simulink model "Copy_2_of_quad_drone"  (R2026a)
settings: Solver=ode4  StopTime=110
values from neighbouring files (symbols this model uses):
  accel_bias_init = [0.05; -0.03; 0.04]    [drone_params.m]    (also in new_drone_params.m)
  accel_drift_std = 0.0001    [drone_params.m]    (also in new_drone_params.m)
  accel_noise_std = 0.007    [drone_params.m]    (also in new_drone_params.m)
  circle_alt = -10    [drone_params.m]    (also in new_drone_params.m)
  circle_center_x = 0    [drone_params.m]    (also in new_drone_params.m)
  circle_center_y = 0    [drone_params.m]    (also in new_drone_params.m)
  circle_radius = 15    [drone_params.m]    (also in new_drone_params.m)
  circle_speed = 1.0    (= 1)    [drone_params.m]    (also in new_drone_params.m)
  g = 9.81    [drone_params.m]    (also in new_drone_params.m)
  gyro_bias_init = [0.002; -0.001; 0.003]    [drone_params.m]    (also in new_drone_params.m)
  gyro_drift_std = 0.0001    [drone_params.m]    (also in new_drone_params.m)
  gyro_noise_std = 0.005    [drone_params.m]    (also in new_drone_params.m)
  kD = 1.5e-7    (= 1.5e-07)    [drone_params.m]    (also in new_drone_params.m)
  Kd_att = [3.5; 3.5; 2]    [drone_params.m]    (also in new_drone_params.m)
  Kd_pos = [0.8; 1.2; 1.8]    [drone_params.m]    (also in new_drone_params.m)
  Kp_att = [6; 6; 4]    [drone_params.m]    (also in new_drone_params.m)
  Kp_pos = [0.5; 0.5; 1.0]    [drone_params.m]    (also in new_drone_params.m)
  kT = 1.2e-5    (= 1.2e-05)    [drone_params.m]    (also in new_drone_params.m)
  L = 0.25    [drone_params.m]    (also in new_drone_params.m; pnp_solver.m = pts_3d(i,:)')
  landmarks_3D = [city_landmarks; road_pts; light_pts; tree_pts; ground_pts]    [drone_params.m]    (also in initialize_map.m = zeros(500, 3); new_drone_params.m)
  m = 1.5    [drone_params.m]    (also in new_drone_params.m)
  num_landmarks = size(landmarks_3D, 1)    [drone_params.m]    (also in new_drone_params.m)
  P0 = K * [eye(3), zeros(3,1)]    [demo_vo_real_world.m]    (also in drone_params.m = diag([0.1, 0.1, 0.1,             0.1, 0.1, 0.1,             ; initialize_map.m; new_drone_params.m = diag([0.1, 0.1, 0.1,             0.1, 0.1, 0.1,             )
  Q_ekf = diag([1e-4, 1e-4, 1e-4,                1e-3, 1e-3, 1e-3,                1e-4, 1e-4, 1e-4,                1e-9, 1e-9, 1e-9,                1e-9, 1e-9, 1e-9])    [drone_params.m]    (also in new_drone_params.m)
  R_cam_body = [0 1 0; 0 0 1; 1 0 0]    [drone_params.m]    (also in generate_camera_frame.m; new_drone_params.m)
  R_ekf = diag([0.08^2, 0.08^2, 0.08^2,      0.05^2, 0.05^2, 0.05^2])    [drone_params.m]    (also in new_drone_params.m)
  takeoff_time = 12    [drone_params.m]    (also in new_drone_params.m)
  Ts = 0.001    [drone_params.m]    (also in new_drone_params.m)
  x0_ekf = Simulink.Parameter    [drone_params.m]
libraries: simulink x1, matrix_library x1
settings Model: Creator=Intern2  LastModifiedBy=Intern2
settings RTWCC: Toolchain=Microsoft Visual C++ 2022 v17.0 | nmake (64-bit Windows)

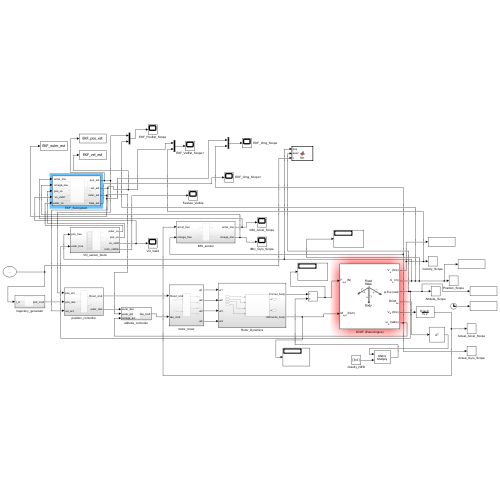
[thumbnail: Simulink's stored preview of the top-level diagram]
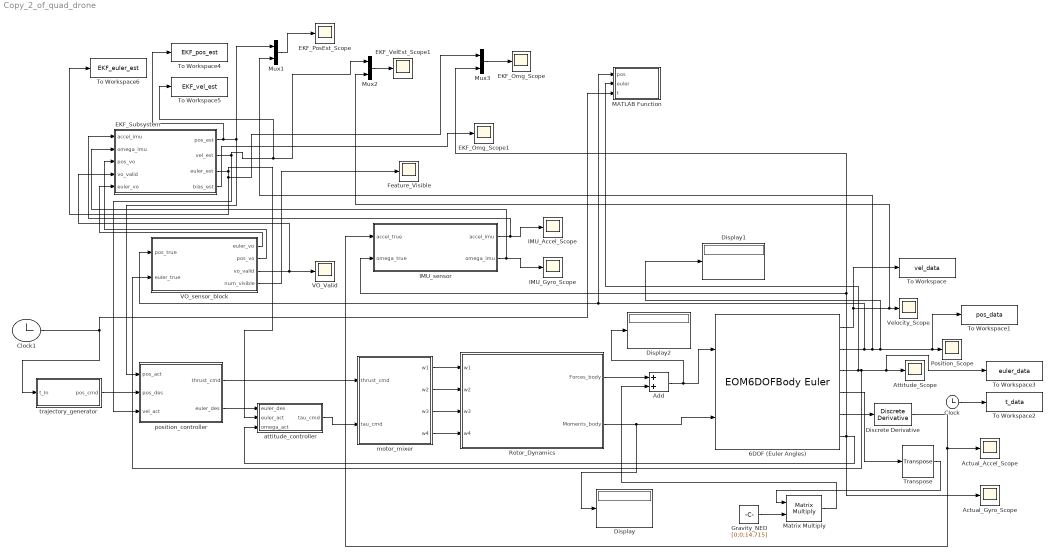
== system Copy_2_of_quad_drone ==
  6DOF (Euler Angles) : EOM6DOFBodyEuler  xme_0=pos_0  Vm_0=vel_0  eul_0=euler_0  pm_0=omega_0  mass_0=m  inertia=I_body
  Actual_Accel_Scope : Scope
      settings: ActiveDisplayYMinimum=-0.50165246590945589  ActiveDisplayYMaximum=0.65110460381560342  DataLoggingVariableName=ScopeData5
  Actual_Gyro_Scope : Scope
      settings: ActiveDisplayYMinimum=-0.42328851957372776  ActiveDisplayYMaximum=0.43797939700166927  DataLoggingVariableName=ScopeData6
  Add : Sum
  Attitude_Scope : Scope
      settings: ActiveDisplayYMinimum=-4.9243572148197217  ActiveDisplayYMaximum=6.6592750571240353  DataLoggingVariableName=ScopeData2
  Clock : Clock
  Clock1 : Clock
  Discrete Derivative : simulink/Discrete/Discrete Derivative  gainval=1.0  ICPrevScaledInput=0.0  OutMin=[]  OutMax=[]  OutDataType=fixdt(1, 16)  OutScaling=2^-10  DoSatur=off
  Display : Display
  Display1 : Display
  Display2 : Display
  EKF_Omg_Scope : Scope
      settings: ActiveDisplayYMinimum=-2.2293879743404958  ActiveDisplayYMaximum=4.7882717816873033  DataLoggingVariableName=ScopeData7
  EKF_Omg_Scope1 : Scope
      settings: ActiveDisplayYMinimum=-1.3068915384977462  ActiveDisplayYMaximum=2.7961887787070889  DataLoggingVariableName=ScopeData12
  EKF_PosEst_Scope : Scope
      settings: ActiveDisplayYMinimum=-40.340225147438069  ActiveDisplayYMaximum=49.360325650117439  DataLoggingVariableName=ScopeData10
  EKF_Subsystem : Subsystem
  EKF_VelEst_Scope1 : Scope
      settings: ActiveDisplayYMinimum=-3.7944004770804414  ActiveDisplayYMaximum=3.6966528557513043  DataLoggingVariableName=ScopeData11
  Feature_Visible : Scope
      settings: ActiveDisplayYMinimum=-641.958251221389  ActiveDisplayYMaximum=573.11142304309487  DataLoggingVariableName=ScopeData8
  Gravity_NED : Constant  Value=[0;0;14.715]
  IMU_Accel_Scope : Scope
      settings: ActiveDisplayYMinimum=-1.9727778311938033  ActiveDisplayYMaximum=2.0010412781388083  DataLoggingVariableName=ScopeData3
  IMU_Gyro_Scope : Scope
      settings: ActiveDisplayYMinimum=-0.092596809772179461  ActiveDisplayYMaximum=0.10856975643800111  DataLoggingVariableName=ScopeData4
  IMU_sensor : Subsystem
  MATLAB Function : MATLAB Function  TreatAsAtomicUnit=on
  Matrix Multiply : Product  Multiplication=Matrix(*)
  Mux1 : Mux  Inputs=2
  Mux2 : Mux  Inputs=2
  Mux3 : Mux  Inputs=2
  Position_Scope : Scope
      settings: ActiveDisplayYMinimum=-93.002014723178334  ActiveDisplayYMaximum=157.03895632222842
  Rotor_Dynamics : Subsystem
  To Workspace : ToWorkspace  VariableName=vel_data  SampleTime=-1
  To Workspace1 : ToWorkspace  VariableName=pos_data  SampleTime=-1
  To Workspace2 : ToWorkspace  VariableName=t_data  SampleTime=-1
  To Workspace3 : ToWorkspace  VariableName=euler_data  SampleTime=-1
  To Workspace4 : ToWorkspace  VariableName=EKF_pos_est  SampleTime=-1
  To Workspace5 : ToWorkspace  VariableName=EKF_vel_est  SampleTime=-1
  To Workspace6 : ToWorkspace  VariableName=EKF_euler_est  SampleTime=-1
  Transpose : matrix_library/Transpose
  VO_Valid : Scope
      settings: ActiveDisplayYMinimum=-4.4680085557439737  ActiveDisplayYMaximum=3.9129303872615759  DataLoggingVariableName=ScopeData9
  VO_sensor_block : Subsystem
  Velocity_Scope : Scope
      settings: ActiveDisplayYMinimum=-4.9122078126709239  ActiveDisplayYMaximum=7.6687377025465322
  attitude_controller : Subsystem
  motor_mixer : Subsystem
  position_controller : Subsystem
  trajectory_generator : Subsystem
  wires:
  6DOF (Euler Angles)/3 -> VO_sensor_block/2(euler_true), To Workspace3/1, Attitude_Scope/1, MATLAB Function/2(euler)
  Clock/1 -> To Workspace2/1
  Rotor_Dynamics/2(Moments_body) -> 6DOF (Euler Angles)/2, Display/1
  motor_mixer/1(w1) -> Rotor_Dynamics/1(w1)
  motor_mixer/2(w2) -> Rotor_Dynamics/2(w2)
  motor_mixer/3(w3) -> Rotor_Dynamics/3(w3)
  motor_mixer/4(w4) -> Rotor_Dynamics/4(w4)
  attitude_controller/1(tau_cmd) -> motor_mixer/2(tau_cmd)
  trajectory_generator/1(pos_cmd) -> position_controller/2(pos_des)
  position_controller/2(euler_des) -> attitude_controller/1(euler_des)
  position_controller/1(thrust_cmd) -> motor_mixer/1(thrust_cmd)
  6DOF (Euler Angles)/2 -> MATLAB Function/1(pos), VO_sensor_block/1(pos_true), To Workspace1/1, Position_Scope/1, Display1/1, Mux1/2
  6DOF (Euler Angles)/4 -> Transpose/1
  Transpose/1 -> Matrix Multiply/1
  Gravity_NED/1 -> Matrix Multiply/2
  Rotor_Dynamics/1(Forces_body) -> Add/1
  Matrix Multiply/1 -> Add/2
  Add/1 -> Display2/1, 6DOF (Euler Angles)/1
  Clock1/1 -> MATLAB Function/3(t), trajectory_generator/1(t_In)
  6DOF (Euler Angles)/6 -> Mux3/2, IMU_sensor/2(omega_true), attitude_controller/3(omega_act), Actual_Gyro_Scope/1
  6DOF (Euler Angles)/5 -> Discrete Derivative/1
  Discrete Derivative/1 -> Actual_Accel_Scope/1, IMU_sensor/1(accel_true)
  IMU_sensor/1(accel_imu) -> EKF_Subsystem/1(" accel_imu"), IMU_Accel_Scope/1
  IMU_sensor/2(omega_imu) -> EKF_Subsystem/2(" omega_imu"), IMU_Gyro_Scope/1
  VO_sensor_block/4(num_visible) -> Feature_Visible/1
  Mux2/1 -> EKF_VelEst_Scope1/1
  EKF_Subsystem/3(euler_est) -> attitude_controller/2(euler_act), To Workspace6/1, Mux3/1
  Mux3/1 -> EKF_Omg_Scope/1
  EKF_Subsystem/2(vel_est) -> To Workspace5/1, Mux2/1, position_controller/3(vel_act)
  EKF_Subsystem/1(pos_est) -> To Workspace4/1, Mux1/1, position_controller/1(pos_act)
  EKF_Subsystem/4(bias_est) -> EKF_Omg_Scope1/1
  6DOF (Euler Angles)/1 -> To Workspace/1, Mux2/2, Velocity_Scope/1
  VO_sensor_block/3(vo_valid) -> EKF_Subsystem/4("  vo_valid"), VO_Valid/1
  VO_sensor_block/1(euler_vo) -> EKF_Subsystem/5(euler_vo)
  VO_sensor_block/2(pos_vo) -> EKF_Subsystem/3(" pos_vo")
  Mux1/1 -> EKF_PosEst_Scope/1

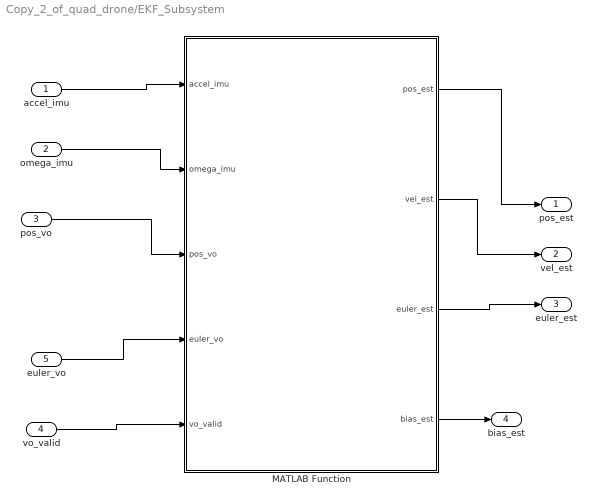
== system Copy_2_of_quad_drone/EKF_Subsystem ==
  " accel_imu" : Inport
  " omega_imu" : Inport  Port=2
  " pos_vo" : Inport  Port=3
  "  vo_valid" : Inport  Port=4
  euler_vo : Inport  Port=5
  MATLAB Function : MATLAB Function  TreatAsAtomicUnit=on
  pos_est : Outport  PortDimensions=[3,1]
  vel_est : Outport  Port=2  PortDimensions=[3,1]
  euler_est : Outport  Port=3  PortDimensions=[3,1]
  bias_est : Outport  Port=4  PortDimensions=[3,1]
  wires:
  MATLAB Function/1(pos_est) -> pos_est/1
  MATLAB Function/2(vel_est) -> vel_est/1
  MATLAB Function/3(euler_est) -> euler_est/1
  " accel_imu"/1 -> MATLAB Function/1(accel_imu)
  " omega_imu"/1 -> MATLAB Function/2(omega_imu)
  " pos_vo"/1 -> MATLAB Function/3(pos_vo)
  "  vo_valid"/1 -> MATLAB Function/5(vo_valid)
  MATLAB Function/4(bias_est) -> bias_est/1
  euler_vo/1 -> MATLAB Function/4(euler_vo)

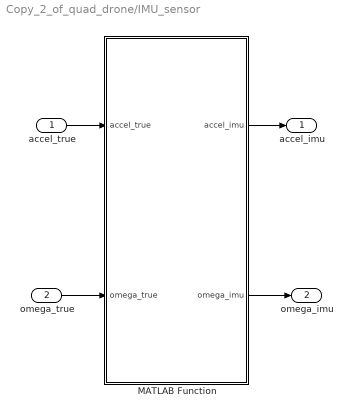
== system Copy_2_of_quad_drone/IMU_sensor ==
  accel_true : Inport
  omega_true : Inport  Port=2
  MATLAB Function : MATLAB Function  TreatAsAtomicUnit=on
  accel_imu : Outport
  omega_imu : Outport  Port=2
  wires:
  accel_true/1 -> MATLAB Function/1(accel_true)
  omega_true/1 -> MATLAB Function/2(omega_true)
  MATLAB Function/1(accel_imu) -> accel_imu/1
  MATLAB Function/2(omega_imu) -> omega_imu/1

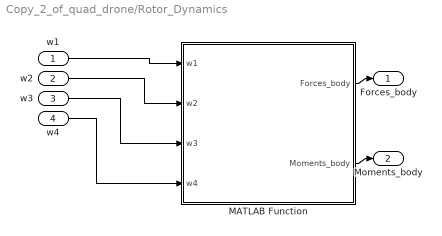
== system Copy_2_of_quad_drone/Rotor_Dynamics ==
  w1 : Inport
  w2 : Inport  Port=2
  w3 : Inport  Port=3
  w4 : Inport  Port=4
  MATLAB Function : MATLAB Function  TreatAsAtomicUnit=on
  Forces_body : Outport
  Moments_body : Outport  Port=2
  wires:
  w1/1 -> MATLAB Function/1(w1)
  w2/1 -> MATLAB Function/2(w2)
  w3/1 -> MATLAB Function/3(w3)
  w4/1 -> MATLAB Function/4(w4)
  MATLAB Function/1(Forces_body) -> Forces_body/1
  MATLAB Function/2(Moments_body) -> Moments_body/1

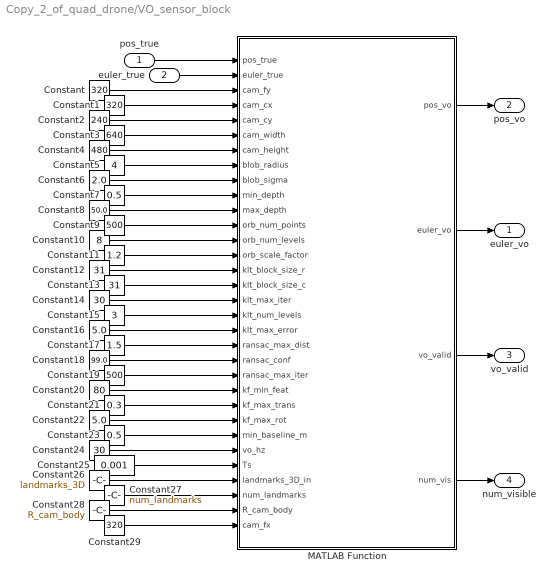
== system Copy_2_of_quad_drone/VO_sensor_block ==
  pos_true : Inport
  euler_true : Inport  Port=2
  Constant : Constant  Value=320
  Constant1 : Constant  Value=320
  Constant10 : Constant  Value=8
  Constant11 : Constant  Value=1.2
  Constant12 : Constant  Value=31
  Constant13 : Constant  Value=31
  Constant14 : Constant  Value=30
  Constant15 : Constant  Value=3
  Constant16 : Constant  Value=5.0
  Constant17 : Constant  Value=1.5
  Constant18 : Constant  Value=99.0
  Constant19 : Constant  Value=500
  Constant2 : Constant  Value=240
  Constant20 : Constant  Value=80
  Constant21 : Constant  Value=0.3
  Constant22 : Constant  Value=5.0
  Constant23 : Constant  Value=0.5
  Constant24 : Constant  Value=30
  Constant25 : Constant  Value=0.001
  Constant26 : Constant  Value=landmarks_3D
  Constant27 : Constant  Value=num_landmarks
  Constant28 : Constant  Value=R_cam_body
  Constant29 : Constant  Value=320
  Constant3 : Constant  Value=640
  Constant4 : Constant  Value=480
  Constant5 : Constant  Value=4
  Constant6 : Constant  Value=2.0
  Constant7 : Constant  Value=0.5
  Constant8 : Constant  Value=50.0
  Constant9 : Constant  Value=500
  MATLAB Function : MATLAB Function  TreatAsAtomicUnit=on
  euler_vo : Outport
  pos_vo : Outport  Port=2
  vo_valid : Outport  Port=3
  num_visible : Outport  Port=4
  wires:
  MATLAB Function/2(euler_vo) -> euler_vo/1
  pos_true/1 -> MATLAB Function/1(pos_true)
  euler_true/1 -> MATLAB Function/2(euler_true)
  MATLAB Function/1(pos_vo) -> pos_vo/1
  MATLAB Function/3(vo_valid) -> vo_valid/1
  MATLAB Function/4(num_vis) -> num_visible/1
  Constant/1 -> MATLAB Function/3(cam_fy)
  Constant1/1 -> MATLAB Function/4(cam_cx)
  Constant2/1 -> MATLAB Function/5(cam_cy)
  Constant3/1 -> MATLAB Function/6(cam_width)
  Constant4/1 -> MATLAB Function/7(cam_height)
  Constant5/1 -> MATLAB Function/8(blob_radius)
  Constant6/1 -> MATLAB Function/9(blob_sigma)
  Constant7/1 -> MATLAB Function/10(min_depth)
  Constant8/1 -> MATLAB Function/11(max_depth)
  Constant9/1 -> MATLAB Function/12(orb_num_points)
  Constant10/1 -> MATLAB Function/13(orb_num_levels)
  Constant11/1 -> MATLAB Function/14(orb_scale_factor)
  Constant12/1 -> MATLAB Function/15(klt_block_size_r)
  Constant13/1 -> MATLAB Function/16(klt_block_size_c)
  Constant14/1 -> MATLAB Function/17(klt_max_iter)
  Constant15/1 -> MATLAB Function/18(klt_num_levels)
  Constant16/1 -> MATLAB Function/19(klt_max_error)
  Constant17/1 -> MATLAB Function/20(ransac_max_dist)
  Constant18/1 -> MATLAB Function/21(ransac_conf)
  Constant19/1 -> MATLAB Function/22(ransac_max_iter)
  Constant20/1 -> MATLAB Function/23(kf_min_feat)
  Constant21/1 -> MATLAB Function/24(kf_max_trans)
  Constant22/1 -> MATLAB Function/25(kf_max_rot)
  Constant23/1 -> MATLAB Function/26(min_baseline_m)
  Constant24/1 -> MATLAB Function/27(vo_hz)
  Constant25/1 -> MATLAB Function/28(Ts)
  Constant26/1 -> MATLAB Function/29(landmarks_3D_in)
  Constant27/1 -> MATLAB Function/30(num_landmarks)
  Constant28/1 -> MATLAB Function/31(R_cam_body)
  Constant29/1 -> MATLAB Function/32(cam_fx)

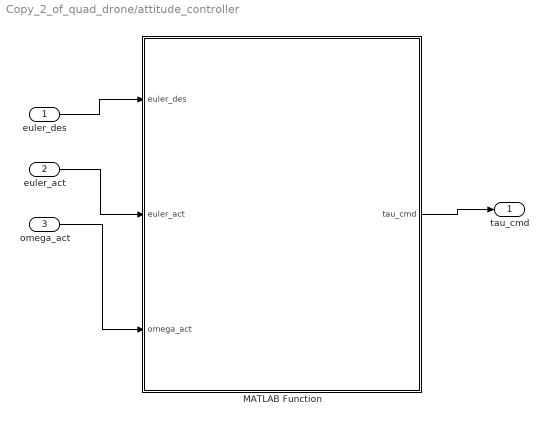
== system Copy_2_of_quad_drone/attitude_controller ==
  euler_des : Inport
  euler_act : Inport  Port=2
  omega_act : Inport  Port=3
  MATLAB Function : MATLAB Function  TreatAsAtomicUnit=on
  tau_cmd : Outport
  wires:
  MATLAB Function/1(tau_cmd) -> tau_cmd/1
  euler_des/1 -> MATLAB Function/1(euler_des)
  euler_act/1 -> MATLAB Function/2(euler_act)
  omega_act/1 -> MATLAB Function/3(omega_act)

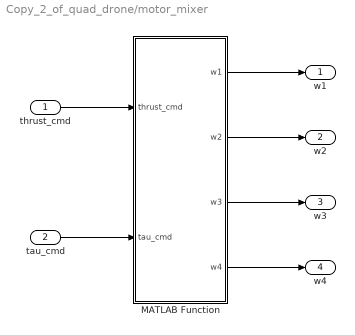
== system Copy_2_of_quad_drone/motor_mixer ==
  thrust_cmd : Inport
  tau_cmd : Inport  Port=2
  MATLAB Function : MATLAB Function  TreatAsAtomicUnit=on
  w1 : Outport
  w2 : Outport  Port=2
  w3 : Outport  Port=3
  w4 : Outport  Port=4
  wires:
  tau_cmd/1 -> MATLAB Function/2(tau_cmd)
  thrust_cmd/1 -> MATLAB Function/1(thrust_cmd)
  MATLAB Function/4(w4) -> w4/1
  MATLAB Function/3(w3) -> w3/1
  MATLAB Function/2(w2) -> w2/1
  MATLAB Function/1(w1) -> w1/1

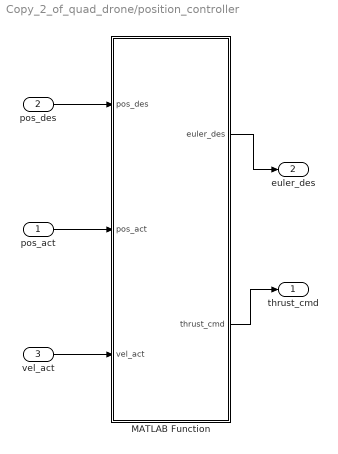
== system Copy_2_of_quad_drone/position_controller ==
  pos_act : Inport
  pos_des : Inport  Port=2
  vel_act : Inport  Port=3
  MATLAB Function : MATLAB Function  TreatAsAtomicUnit=on
  thrust_cmd : Outport
  euler_des : Outport  Port=2
  wires:
  pos_act/1 -> MATLAB Function/2(pos_act)
  pos_des/1 -> MATLAB Function/1(pos_des)
  vel_act/1 -> MATLAB Function/3(vel_act)
  MATLAB Function/1(euler_des) -> euler_des/1
  MATLAB Function/2(thrust_cmd) -> thrust_cmd/1

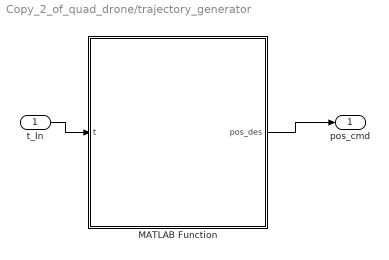
== system Copy_2_of_quad_drone/trajectory_generator ==
  t_In : Inport
  MATLAB Function : MATLAB Function  TreatAsAtomicUnit=on
  pos_cmd : Outport
  wires:
  MATLAB Function/1(pos_des) -> pos_cmd/1
  t_In/1 -> MATLAB Function/1(t)

== matlab function Copy_2_of_quad_drone/IMU_sensor/MATLAB Function ==
  settings: updateMethod=DISCRETE  sampleTime=0.001
  data: accel_true input; accel_imu output; omega_true input; omega_imu output; accel_noise_std parameter; accel_bias_init parameter; accel_drift_std parameter; gyro_noise_std parameter; gyro_bias_init parameter; gyro_drift_std parameter
function [accel_imu, omega_imu] = imu_sensor(accel_true, omega_true, ...
    accel_noise_std, accel_bias_init, accel_drift_std, ...
gyro_noise_std, gyro_bias_init, gyro_drift_std)
%#codegen

persistent accel_bias gyro_bias;

if isempty(accel_bias)
    accel_bias = accel_bias_init;
    gyro_bias  = gyro_bias_init;
end

% Bias random walk (drift)
accel_bias = accel_bias + accel_drift_std * randn(3,1);
gyro_bias  = gyro_bias  + gyro_drift_std  * randn(3,1);

% Add noise + bias to true measurements
accel_imu = accel_true + accel_bias + accel_noise_std * randn(3,1);
omega_imu = omega_true + gyro_bias  + gyro_noise_std  * randn(3,1);
end

== matlab function Copy_2_of_quad_drone/MATLAB Function ==
  data: pos input size=[3,1]; euler input size=[3,1]; t input size=1
function fcn(pos, euler, t)
    coder.extrinsic('live_flight_update');
    live_flight_update(pos, euler, t);
end

== matlab function Copy_2_of_quad_drone/EKF_Subsystem/MATLAB Function ==
  settings: updateMethod=DISCRETE  sampleTime=0.001
  data: accel_imu input; pos_est output size=[3 1]; omega_imu input; pos_vo input size=[3,1]; euler_vo input size=[3,1]; vo_valid input size=1; vel_est output size=[3 1]; euler_est output size=[3 1]; P0 parameter size=[15,15]; Q_ekf parameter size=[15,15]; R_ekf parameter size=[6,6]; x0_ekf parameter size=[15,1]; Ts parameter; bias_est output size=[3,1]
function [pos_est, vel_est, euler_est, bias_est] = ekf(accel_imu, omega_imu, ...
    pos_vo, euler_vo, vo_valid, P0, Q_ekf, R_ekf, x0_ekf, Ts)
%#codegen
% 15-State EKF — fuses IMU (1kHz) with VO pose (30Hz)
%
% State: [pos(3); vel(3); euler(3); accel_bias(3); gyro_bias(3)]
% VO Measurements: [pos(3); euler(3)] = 6 measurements

persistent x P;
if isempty(x)
    x = x0_ekf;
    P = P0;
end

%% BIAS CORRECTION
accel_corrected = accel_imu - x(10:12);
omega_corrected = omega_imu - x(13:15);

%% ROTATION MATRIX
roll = x(7); pitch = x(8); yaw = x(9);
cr = cos(roll);  sr = sin(roll);
cp = cos(pitch); sp = sin(pitch);
cy = cos(yaw);   sy = sin(yaw);

R_be = [cy*cp,  cy*sp*sr - sy*cr,  cy*sp*cr + sy*sr;
        sy*cp,  sy*sp*sr + cy*cr,  sy*sp*cr - cy*sr;
        -sp,    cp*sr,              cp*cr];

%% PREDICT — State
accel_earth = R_be * accel_corrected;

x(1:3) = x(1:3) + Ts * x(4:6);
x(4:6) = x(4:6) + Ts * accel_earth;
x(7:9) = x(7:9) + Ts * omega_corrected;

%% PREDICT — Covariance
F = eye(15);
F(1,4) = Ts;  F(2,5) = Ts;  F(3,6) = Ts;
F(4:6, 10:12) = -Ts * R_be;
F(7,13) = -Ts;  F(8,14) = -Ts;  F(9,15) = -Ts;

P = F * P * F' + Q_ekf;

%% UPDATE — VO Pose (position + orientation, 6 measurements)
if vo_valid > 0.5
    H = zeros(6, 15);
    H(1,1) = 1;  H(2,2) = 1;  H(3,3) = 1;   % position
    H(4,7) = 1;  H(5,8) = 1;  H(6,9) = 1;   % euler

    z_meas = [pos_vo; euler_vo];
    z_pred = [x(1:3); x(7:9)];
    innov  = z_meas - z_pred;

    S_mat = H * P * H' + R_ekf;
    K     = P * H' / S_mat;

    x = x + K * innov;
    P = (eye(15) - K * H) * P;
end

pos_est   = x(1:3);
vel_est   = x(4:6);
euler_est = x(7:9);
bias_est  = x(10:12);
end

== matlab function Copy_2_of_quad_drone/VO_sensor_block/MATLAB Function ==
  settings: updateMethod=DISCRETE  sampleTime=0.001
  data: pos_true input size=[3,1]; pos_vo output size=[3,1]; euler_true input size=[3,1]; cam_fy input; cam_cx input; cam_cy input; cam_width input; cam_height input; blob_radius input; blob_sigma input; min_depth input; max_depth input; orb_num_points input; orb_num_levels input; orb_scale_factor input; klt_block_size_r input; klt_block_size_c input; klt_max_iter input; klt_num_levels input; klt_max_error input; ransac_max_dist input; ransac_conf input; ransac_max_iter input; kf_min_feat input; kf_max_trans input; kf_max_rot input; min_baseline_m input; vo_hz input; Ts input; landmarks_3D_in input; num_landmarks input; R_cam_body input; euler_vo output size=[3,1]; vo_valid output; num_vis output; cam_fx input
function [pos_vo, euler_vo, vo_valid, num_vis] = vo_new_block(...
           pos_true, euler_true, ...
           cam_fy, cam_cx, cam_cy, ...
           cam_width, cam_height, ...
           blob_radius, blob_sigma, ...
           min_depth, max_depth, ...
           orb_num_points, orb_num_levels, orb_scale_factor, ...
           klt_block_size_r, klt_block_size_c, ...
           klt_max_iter, klt_num_levels, klt_max_error, ...
           ransac_max_dist, ransac_conf, ransac_max_iter, ...
           kf_min_feat, kf_max_trans, kf_max_rot, ...
           min_baseline_m, vo_hz, Ts, ...
           landmarks_3D_in, num_landmarks, R_cam_body, cam_fx)
%#codegen
% VO_NEW_BLOCK  Full VO pipeline (Module 1+2+3) for Simulink
% Inputs:  true pos/euler from 6-DOF block (frame generation only)
% Outputs: ESTIMATED pos/euler from VO pipeline feeds EKF
%
% kp_kf stores MAP PROJECTIONS into keyframe (not ORB keypoints)
% guarantees correct 2D-3D correspondence via KLT tracking

persistent counter initialized init_checking ...
           frame_prev kp_kf pos_kf euler_kf frame_kf ...
           map_3d map_size ...
           last_pos last_euler ...
           pos_0 euler_0 frame_0 kp_0;

if isempty(counter)
    counter       = int32(0);
    initialized   = false;
    init_checking = false;
    frame_prev    = zeros(480, 640, 'uint8');
    frame_kf      = zeros(480, 640, 'uint8');
    frame_0       = zeros(480, 640, 'uint8');
    kp_kf         = zeros(2000, 2);
    kp_0          = zeros(500,  2);
    pos_kf        = zeros(3, 1);
    euler_kf      = zeros(3, 1);
    map_3d        = zeros(2000, 3);
    map_size      = int32(0);
    last_pos      = zeros(3, 1);
    last_euler    = zeros(3, 1);
    pos_0         = zeros(3, 1);
    euler_0       = zeros(3, 1);
end

% ---- Throttle to vo_hz -----------------------------------------
update_interval = int32(round(1.0 / (vo_hz * Ts)));
counter = counter + int32(1);

if counter < update_interval
    pos_vo   = last_pos;
    euler_vo = last_euler;
    vo_valid = double(initialized);
    num_vis  = double(map_size);
    return;
end
counter = int32(0);

% ---- Build parameter structs -----------------------------------
cam_p.fx          = cam_fx;
cam_p.fy          = cam_fy;
cam_p.cx          = cam_cx;
cam_p.cy          = cam_cy;
cam_p.width       = cam_width;
cam_p.height      = cam_height;
cam_p.blob_radius = blob_radius;
cam_p.blob_sigma  = blob_sigma;
cam_p.min_depth   = min_depth;
cam_p.max_depth   = max_depth;

orb_p.num_points   = orb_num_points;
orb_p.num_levels   = orb_num_levels;
orb_p.scale_factor = orb_scale_factor;

klt_p.block_size     = [klt_block_size_r, klt_block_size_c];
klt_p.max_iterations = klt_max_iter;
klt_p.num_levels     = klt_num_levels;
klt_p.max_error      = klt_max_error;

ran_p.max_distance   = ransac_max_dist;
ran_p.confidence     = ransac_conf;
ran_p.max_iterations = ransac_max_iter;

kf_p.min_features    = kf_min_feat;
kf_p.max_translation = kf_max_trans;
kf_p.max_rotation    = kf_max_rot;

landmarks = landmarks_3D_in(1:num_landmarks, :);

% ================================================================
% PHASE A: Waiting for map initialisation
% ================================================================
if ~initialized

    frame_curr = generate_camera_frame(...
        pos_true, euler_true, landmarks', cam_p);

    if ~init_checking
        frame_0    = frame_curr;
        pos_0      = pos_true;
        euler_0    = euler_true;
        kp_temp    = detect_orb_features(frame_0, orb_p);
        n0         = size(kp_temp, 1);
        kp_0       = zeros(500, 2);
        kp_0(1:n0,:) = kp_temp;
        frame_prev    = frame_0;
        frame_kf      = frame_0;
        init_checking = true;

        pos_vo=last_pos; euler_vo=last_euler;
        vo_valid=0; num_vis=0;
        return;
    end

    [ready, dist] = check_baseline(pos_0, pos_true, min_baseline_m);
    if ~ready
        pos_vo=last_pos; euler_vo=last_euler;
        vo_valid=0; num_vis=0;
        return;
    end

    fprintf('[INIT] Baseline ready: %.3fm\n', dist);

    kp_0_active = kp_0(any(kp_0~=0,2), :);
    [kp2, val, ~] = track_klt_features(frame_0, frame_curr, kp_0_active, klt_p);

    if sum(val) >= 8
        [p0, pK, ~, n_in] = ransac_filter(...
            kp_0_active(val,:), kp2(val,:), ran_p);

        if n_in >= 8
            [lm_cam0, ~, ~, ~, ~, ~, ok] = initialize_map(...
    frame_0, frame_curr, p0, pK, pos_0, pos_true, cam_p);
            if ok && size(lm_cam0,1) >= 8
                % Transform lm_cam0 → world NED
                R_be_0 = build_Rec(euler_0, R_cam_body)' * R_cam_body;
                % Simpler: build R_be_0 directly
                roll=euler_0(1); pitch=euler_0(2); yaw=euler_0(3);
                cr=cos(roll); sr=sin(roll); cp=cos(pitch);
                sp=sin(pitch); cy_=cos(yaw); sy_=sin(yaw);
                R_be_0=[cy_*cp, cy_*sp*sr-sy_*cr, cy_*sp*cr+sy_*sr;
                        sy_*cp, sy_*sp*sr+cy_*cr,  sy_*sp*cr-cy_*sr;
                        -sp,    cp*sr,               cp*cr           ];

                n_lm = size(lm_cam0,1);
                for i = 1:n_lm
                    p_body      = R_cam_body' * lm_cam0(i,:)';
                    p_world     = R_be_0 * p_body + pos_0;
                    map_3d(i,:) = p_world';
                end
                map_size = int32(n_lm);

                % Project map into current frame → kp_kf
                kp_kf = project_map_into_frame(...
                    map_3d, n_lm, pos_true, euler_true, ...
                    R_cam_body, cam_fx, cam_fy, cam_cx, cam_cy, ...
                    cam_width, cam_height, min_depth, max_depth);

                pos_kf      = pos_true;
                euler_kf    = euler_true;
                frame_kf    = frame_curr;
                frame_prev  = frame_curr;
                last_pos    = pos_true;
                last_euler  = euler_true;
                initialized = true;

                fprintf('[INIT] Map ready: %i landmarks\n', int32(n_lm));
            end
        end
    end

    pos_vo   = last_pos;
    euler_vo = last_euler;
    vo_valid = 0;
    num_vis  = double(map_size);
    return;
end

% ================================================================
% PHASE B: Map ready — run back-end every VO frame
% ================================================================
frame_curr   = generate_camera_frame(pos_true, euler_true, landmarks', cam_p);
cur_map_size = double(map_size);

% Check active projections WITHOUT slicing kp_kf — keep it fixed-size
n_active = sum(any(kp_kf(1:cur_map_size,:)~=0, 2));
if n_active < 6
    fprintf('[BACKEND] Too few active projections: %i\n', int32(n_active));
    pos_vo=last_pos; euler_vo=last_euler;
    vo_valid=1; num_vis=double(map_size);
    frame_prev = frame_curr;
    return;
end

% Pass the FULL fixed-size kp_kf (2000x2) — run_backend slices internally
[pos_out, euler_out, valid_out, map_3d, map_size, kp_kf] = run_backend(...
    frame_kf, frame_curr, ...
    kp_kf, pos_kf, euler_kf, ...
    pos_true, euler_true, ...
    map_3d, map_size, ...
    cam_p, R_cam_body, ...
    orb_p, klt_p, ran_p, kf_p, ...
    last_pos, last_euler);

if valid_out
    last_pos   = pos_out;
    last_euler = euler_out;

    d_pos   = norm(pos_true  - pos_kf);
    d_euler = norm(euler_true - euler_kf) * 180/pi;

    if d_pos > kf_p.max_translation || d_euler > kf_p.max_rotation

        fprintf('[KF] New keyframe — d_pos=%.2fm  d_euler=%.1fdeg\n', ...
            d_pos, d_euler);

        % Re-project map into current frame
        kp_kf = project_map_into_frame(...
            map_3d, double(map_size), pos_true, euler_true, ...
            R_cam_body, cam_fx, cam_fy, cam_cx, cam_cy, ...
            cam_width, cam_height, min_depth, max_depth);

        pos_kf   = pos_true;
        euler_kf = euler_true;
        frame_kf = frame_curr;
    end
end

frame_prev = frame_curr;
pos_vo     = last_pos;
euler_vo   = last_euler;
vo_valid   = double(valid_out);
num_vis    = double(map_size);
end

== matlab function Copy_2_of_quad_drone/motor_mixer/MATLAB Function ==
  settings: updateMethod=DISCRETE  sampleTime=0.001
  data: thrust_cmd input; w1 output; tau_cmd input; w2 output; w3 output; w4 output; kT parameter; kD parameter; L parameter
function [w1,w2,w3,w4] = motor_mixer(thrust_cmd, tau_cmd, kT, kD, L)
%#codegen
tau_r = tau_cmd(1); tau_p = tau_cmd(2); tau_y = tau_cmd(3);

w1sq = thrust_cmd/(4*kT) - tau_p/(2*kT*L) + tau_y/(4*kD);
w2sq = thrust_cmd/(4*kT) - tau_r/(2*kT*L) - tau_y/(4*kD);
w3sq = thrust_cmd/(4*kT) + tau_p/(2*kT*L) + tau_y/(4*kD);
w4sq = thrust_cmd/(4*kT) + tau_r/(2*kT*L) - tau_y/(4*kD);

w1 = min(sqrt(max(0,w1sq)), 1200);
w2 = min(sqrt(max(0,w2sq)), 1200);
w3 = min(sqrt(max(0,w3sq)), 1200);
w4 = min(sqrt(max(0,w4sq)), 1200);
end

== matlab function Copy_2_of_quad_drone/Rotor_Dynamics/MATLAB Function ==
  settings: updateMethod=DISCRETE  sampleTime=0.001
  data: w1 input; Forces_body output; w2 input; w3 input; w4 input; Moments_body output; kT parameter; kD parameter; L parameter
function [Forces_body, Moments_body] = rotor_dynamics(w1, w2, w3, w4, kT, kD, L)
%#codegen
% Compute forces and moments from 4 rotor speeds
%
% Inputs:
%   w1, w2, w3, w4 — rotor speeds [rad/s]
%   kT — thrust coefficient
%   kD — drag coefficient
%   L  — arm length [m]
%
% Outputs:
%   Forces_body  — [Fx; Fy; Fz] in body frame [N]
%   Moments_body — [L_roll; M_pitch; N_yaw] in body frame [N·m]

    % Total thrust (all rotors push in -Z body direction)
    T = kT * (w1^2 + w2^2 + w3^2 + w4^2);
    
    % Force in body frame (thrust is along -Z body axis)
    Forces_body = [0; 0; -T];
    
    % Moments in body frame
    % Roll  (rotation about X): difference between left and right rotors
    tau_roll  = L * kT * (w4^2 - w2^2);
    
    % Pitch (rotation about Y): difference between front and back rotors
    tau_pitch = L * kT * (w3^2 - w1^2);
    
    % Yaw   (rotation about Z): reaction torque from CW vs CCW rotors
    tau_yaw   = kD * (w1^2 - w2^2 + w3^2 - w4^2);
    
    Moments_body = [tau_roll; tau_pitch; tau_yaw];
end

== matlab function Copy_2_of_quad_drone/attitude_controller/MATLAB Function ==
  settings: updateMethod=DISCRETE  sampleTime=0.001
  data: euler_des input; tau_cmd output; euler_act input; omega_act input; Kp_att parameter; Kd_att parameter
function tau_cmd = attitude_controller(euler_des, euler_act, omega_act, Kp_att, Kd_att)
%#codegen
err     = euler_des - euler_act;
d_err   = -omega_act;
tau_cmd = Kp_att .* err + Kd_att .* d_err;
end

== matlab function Copy_2_of_quad_drone/position_controller/MATLAB Function ==
  settings: updateMethod=DISCRETE  sampleTime=0.001
  data: pos_des input; euler_des output; pos_act input; vel_act input; thrust_cmd output; Kp_pos parameter; Kd_pos parameter; m parameter; g parameter
function [euler_des, thrust_cmd] = position_controller(pos_des, pos_act, vel_act, Kp_pos, Kd_pos, m, g)
%#codegen
err        = pos_des - pos_act;
acc_des    = Kp_pos .* err + Kd_pos .* (-vel_act);

thrust_cmd = m * (g - acc_des(3));
thrust_cmd = max(0, thrust_cmd);

safe_thrust = thrust_cmd / m + 1e-6;

% Clamp BEFORE calling asin — input must be in [-1, 1]
pitch_input = max(-1, min(1,  acc_des(1) / safe_thrust));
roll_input  = max(-1, min(1, -acc_des(2) / safe_thrust));

pitch_des   = asin(pitch_input);
roll_des    = asin(roll_input);

% Also clamp output angle to ±30 degrees for safety
pitch_des = max(-0.52, min(0.52, pitch_des));
roll_des  = max(-0.52, min(0.52, roll_des));

euler_des = [roll_des; pitch_des; 0];
end

== matlab function Copy_2_of_quad_drone/trajectory_generator/MATLAB Function ==
  settings: updateMethod=DISCRETE  sampleTime=0.001
  data: t input; pos_des output size=[3,1]; circle_center_x parameter; circle_center_y parameter; circle_radius parameter; circle_alt parameter; circle_speed parameter; takeoff_time parameter
function pos_des = traj_gen_circle(t, circle_center_x, circle_center_y, ...
    circle_radius, circle_alt, circle_speed, takeoff_time)
%#codegen
% Circular Trajectory Generator
%
% Phase 1 (t < takeoff_time): Vertical climb to altitude
% Phase 2 (t >= takeoff_time): Circular orbit
%
% Circle starts at angle = 0 → pos = [cx + R, cy, alt]
% Orbits counter-clockwise (positive Y first)

% Start position: on the circle at angle 0, on the ground
start_x = circle_center_x + circle_radius;
start_y = circle_center_y;

if t < takeoff_time
    %% PHASE 1: Takeoff — climb vertically from ground to altitude
    frac = t / takeoff_time;
    % Smooth acceleration (sinusoidal profile for smooth climb)
    smooth_frac = 0.5 * (1 - cos(pi * frac));
    
    pos_des = [start_x; ...
               start_y; ...
               circle_alt * smooth_frac];     % climb from 0 to circle_alt
else
    %% PHASE 2: Circular orbit
    omega = circle_speed / circle_radius;     % angular velocity [rad/s]
    theta = omega * (t - takeoff_time);       % angle from start
    
    pos_des = [circle_center_x + circle_radius * cos(theta); ...
               circle_center_y + circle_radius * sin(theta); ...
               circle_alt];
end
end
